simulink model "FeedBackLoop_Effect_VS_OpenLoop"  (R2024a)
settings: Solver=VariableStepAuto  StartTime=0.0  StopTime=10.0  RelTol=1e-3
settings Model: Creator=VICTUS  LastModifiedBy=VICTUS

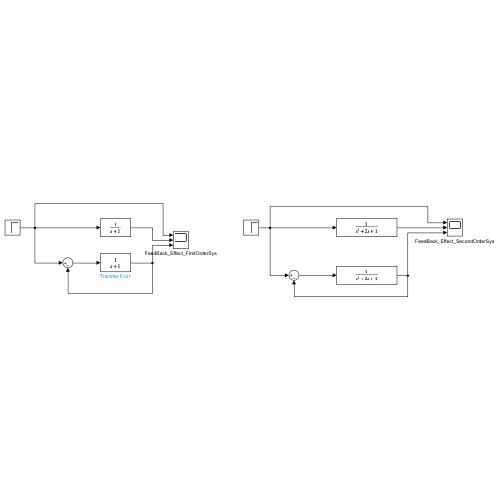
[thumbnail: Simulink's stored preview of the top-level diagram]
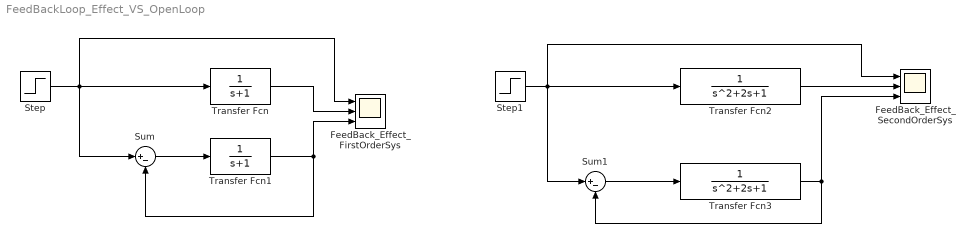
== system FeedBackLoop_Effect_VS_OpenLoop ==
  FeedBack_Effect_FirstOrderSys : Scope  NumInputPorts=3
  FeedBack_Effect_SecondOrderSys : Scope  NumInputPorts=3
  Step : Step  SampleTime=0
  Step1 : Step  SampleTime=0
  Sum : Sum  Inputs=|+-
  Sum1 : Sum  Inputs=|+-
  Transfer Fcn : TransferFcn  Denominator=[1 1]
  Transfer Fcn1 : TransferFcn  Denominator=[1 1]
  Transfer Fcn2 : TransferFcn
  Transfer Fcn3 : TransferFcn
  wires:
  Sum/1 -> Transfer Fcn1/1
  Step/1 -> Sum/1, FeedBack_Effect_FirstOrderSys/1, Transfer Fcn/1
  Transfer Fcn/1 -> FeedBack_Effect_FirstOrderSys/2
  Transfer Fcn1/1 -> FeedBack_Effect_FirstOrderSys/3, Sum/2
  Step1/1 -> Sum1/1, FeedBack_Effect_SecondOrderSys/1, Transfer Fcn2/1
  Transfer Fcn2/1 -> FeedBack_Effect_SecondOrderSys/2
  Transfer Fcn3/1 -> Sum1/2, FeedBack_Effect_SecondOrderSys/3
  Sum1/1 -> Transfer Fcn3/1
